simulink model "Test_Word_Multiplexer_2_to_1"  (Simulink 8.7)
settings: Solver=ode45  StartTime=0.0  StopTime=len  RelTol=1e-3
libraries: Miscellaneous x3, Word_Multiplexers_Lib x1
settings Model: Creator=N  LastModifiedBy=Jozko Mrkvicka
settings DataIOCC: LimitDataPoints=off
settings DebuggingCC: UnderspecifiedInitializationDetection=Simplified  MergeDetectMultiDrivingBlocksExec=error
settings HardwareCC: ProdBitPerPointer=64  ProdLargestAtomicFloat=Float  ProdIntDivRoundTo=Zero  ProdEndianess=LittleEndian  ProdHWDeviceType=Intel->x86-64 (Windows64)
settings ModelReferenceCC: PropagateSignalLabelsOutOfModel=on

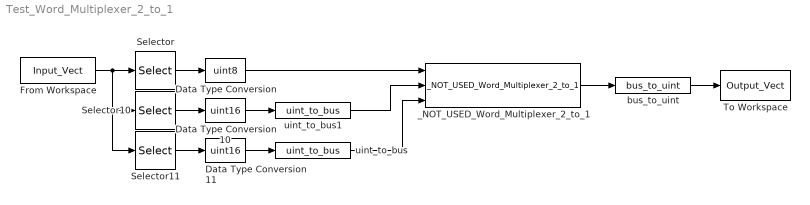
== system Test_Word_Multiplexer_2_to_1 ==
  Data Type Conversion : DataTypeConversion  OutDataTypeStr=uint8
  Data Type Conversion10 : DataTypeConversion  OutDataTypeStr=uint16
  Data Type Conversion11 : DataTypeConversion  OutDataTypeStr=uint16
  From Workspace : FromWorkspace  VariableName=Input_Vect  SampleTime=1  Interpolate=off  OutputAfterFinalValue=Holding final value
  Selector : Selector  IndexMode=Zero-based  InputPortWidth=3  SampleTime=1  IndexOptions=Index vector (dialog)  Indices=0  OutputSizes=1
  Selector10 : Selector  IndexMode=Zero-based  InputPortWidth=3  IndexOptions=Index vector (dialog)  Indices=1  OutputSizes=1
  Selector11 : Selector  IndexMode=Zero-based  InputPortWidth=3  IndexOptions=Index vector (dialog)  Indices=2  OutputSizes=1
  To Workspace : ToWorkspace  VariableName=Output_Vect  SampleTime=1
  _NOT_USED_Word_Multiplexer_2_to_1 : Word_Multiplexers_Lib/Word_Multiplexers_Lib/_NOT_USED_Word_Multiplexer_2_to_1
  bus_to_uint : Miscellaneous/bus_to_uint
  uint_to_bus : Miscellaneous/uint_to_bus
  uint_to_bus1 : Miscellaneous/uint_to_bus
  wires:
  _NOT_USED_Word_Multiplexer_2_to_1/1 -> bus_to_uint/1
  Selector/1 -> Data Type Conversion/1
  Data Type Conversion/1 -> _NOT_USED_Word_Multiplexer_2_to_1/1
  From Workspace/1 -> Selector11/1, Selector10/1, Selector/1
  Selector10/1 -> Data Type Conversion10/1
  Selector11/1 -> Data Type Conversion11/1
  Data Type Conversion10/1 -> uint_to_bus1/1
  Data Type Conversion11/1 -> uint_to_bus/1
  uint_to_bus1/1 -> _NOT_USED_Word_Multiplexer_2_to_1/2
  uint_to_bus/1 -> _NOT_USED_Word_Multiplexer_2_to_1/3
  bus_to_uint/1 -> To Workspace/1
